simulink model "servo_model"  (R2015a)
settings: Solver=ode8  StartTime=0.0  StopTime=50  FixedStep=0.01  RelTol=1e-3
values from neighbouring files (symbols this model uses):
  Beta = 0.00036    [experiment1.mat]    (also in experiment2.mat; experiment3.mat; experiment4.mat; friction_ident.mat = 0.00013)
  f_0 = 0.018    [experiment1.mat]    (also in experiment2.mat; experiment3.mat; experiment4.mat; friction_ident.mat = 0.0018)
  J = 0.001118    [experiment1.mat]    (also in experiment2.mat; experiment3.mat; experiment4.mat; friction_ident.mat = 0.0001118)
  K = 0.053    [experiment1.mat]    (also in experiment2.mat; experiment3.mat; experiment4.mat; friction_ident.mat = 0.0053)
  max_voltage = 13.3    [experiment1.mat]    (also in experiment2.mat; experiment3.mat; experiment4.mat; friction_ident.mat)
  R = 2.71    [experiment1.mat]    (also in experiment2.mat; experiment3.mat; experiment4.mat; friction_ident.mat)
settings Model: Creator=Student  LastModifiedBy=Student

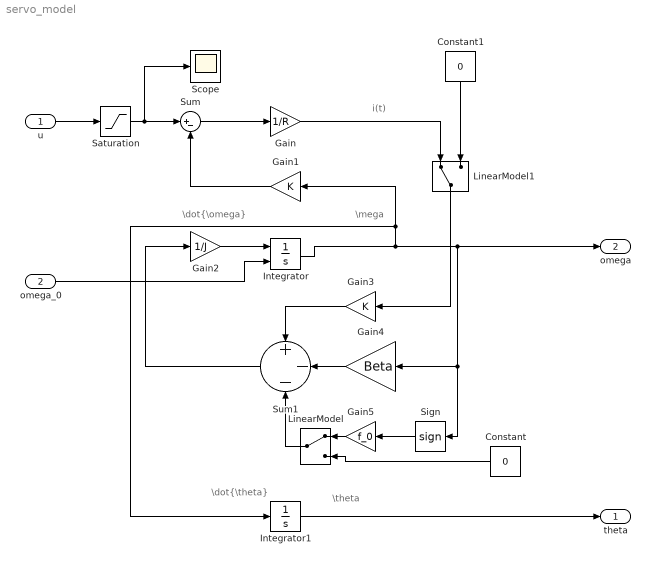
== system servo_model ==
  note: \theta
  note: \dot{\theta}
  note: i(t)
  note: \mega
  note: \dot{\omega}
  u : Inport
  omega_0 : Inport  Port=2
  " LinearModel" : ManualSwitch
  " LinearModel1" : ManualSwitch
  Constant : Constant  Value=0
  Constant1 : Constant  Value=0
  Gain : Gain  Gain=1/R
  Gain1 : Gain  Gain=K
  Gain2 : Gain  Gain=1/J
  Gain3 : Gain  Gain=K
  Gain4 : Gain  Gain=Beta
  Gain5 : Gain  Gain=f_0
  Integrator : Integrator  InitialConditionSource=external  InitialCondition=140
  Integrator1 : Integrator
  Saturation : Saturate  UpperLimit=max_voltage  LowerLimit=-max_voltage
  Scope : Scope
  Sign : Signum
  Sum : Sum  Inputs=|+-
  Sum1 : Sum  Inputs=+--
  theta : Outport
  omega : Outport  Port=2
  wires:
  Gain1/1 -> Sum/2
  Sum/1 -> Gain/1
  Gain2/1 -> Integrator/1
  Gain3/1 -> Sum1/1
  Gain4/1 -> Sum1/2
  Sign/1 -> Gain5/1
  Sum1/1 -> Gain2/1
  Integrator/1 -> Gain1/1, Integrator1/1, omega/1, Sign/1, Gain4/1
  Integrator1/1 -> theta/1
  u/1 -> Saturation/1
  " LinearModel"/1 -> Sum1/3
  Gain5/1 -> " LinearModel"/1
  Constant/1 -> " LinearModel"/2
  Saturation/1 -> Scope/1, Sum/1
  omega_0/1 -> Integrator/2
  Gain/1 -> " LinearModel1"/1
  " LinearModel1"/1 -> Gain3/1
  Constant1/1 -> " LinearModel1"/2
